simulink model "problem2"  (R2020b)
settings: Solver=VariableStepAuto  StartTime=0.0  StopTime=10.0  RelTol=1e-3
settings Model: Creator=Nitin  LastModifiedBy=Nitin

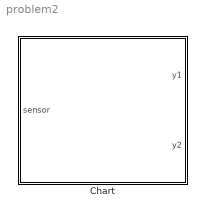
== system problem2 ==
  Chart : Stateflow chart  TreatAsAtomicUnit=on

== stateflow chart problem2/Chart ==
  state Stop
    y1=Red;
    y2=Green;
  state StopforTraffic
    y1=Red;
    y2=Green;
  state StoptoGo
    y1=Red;
    y2=Yellow;
  state GotoStop
    y1=Yellow;
    y2=Red;
  state Go
    y1=Green;
    y2=Red;
  (default) -> Stop
  Stop -> StopforTraffic : after(20,tick)
  StopforTraffic -> StoptoGo : [sensor]
  GotoStop -> Stop : after(3,tick)
  StoptoGo -> Go : after(3,tick)
  Go -> GotoStop : after(10,tick)
  data: sensor input; y1 output; y2 output; Green constant double =3; Red constant double =1; Yellow constant double =2
